simulink model "stuPlutoRx"  (R2021a)
settings: Solver=VariableStepAuto  StartTime=0.0  StopTime=2  RelTol=1e-3
undefined symbols (not defined in the file or in its folder): designMultirateFIR, Fs, ip, usb
libraries: plutoradiolib x1, dsparch4 x1, dspmlti4 x1, dspfdesign x1, dspsrcs4 x1
settings Model: Creator=dm  LastModifiedBy=timingyang
settings SolverCC: AlgebraicLoopSolver=TrustRegion

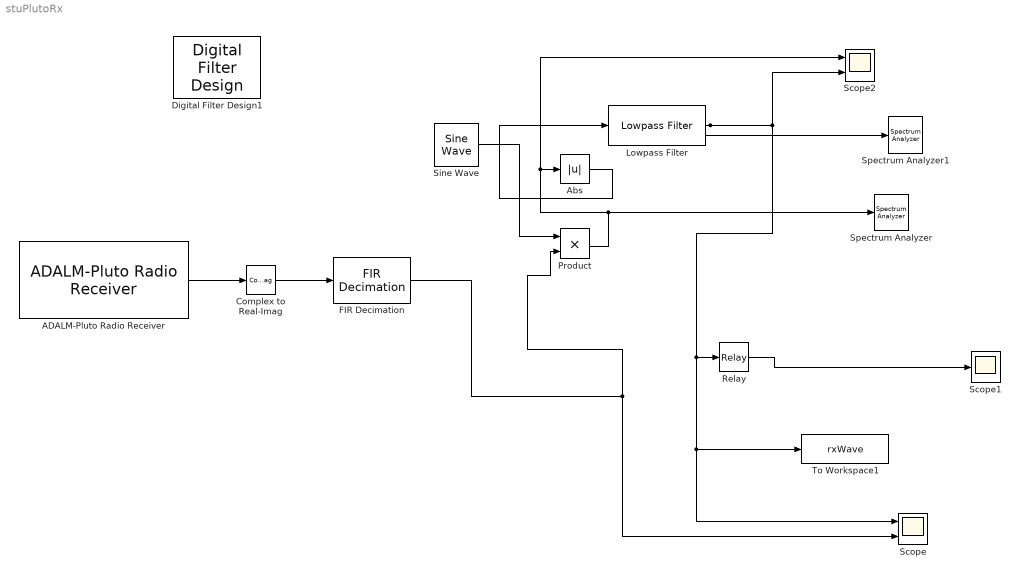
== system stuPlutoRx ==
  ADALM-Pluto Radio Receiver : plutoradiolib/ADALM-Pluto Radio Receiver  RadioID=usb:0  uri=ip:10.0.0.200  CenterFrequencySource=Dialog  CenterFrequency=915.432e6  GainSource=AGC Slow Attack  GainSourceBlock=AGC Slow Attack  Gain=10  ChannelMapping=1  BasebandSampleRate=1e6  OutputDataType=double  SamplesPerFrame=2e4  OverflowOutputPort=off  EnableBurstMode=off  NumFramesInBurst=1  ShowAdvancedProperties=off  UseCustomFilter=off  filtPathRates=[737280000 11520000 3840000 1920000 960000 240000]  filtCoefficients=[-192 82 85 -215 228 -102 -110 290 -318 145 160 -426 471 -215 -238 633 -697 318 349 -923 1009 -457 -498 1309 -1423 640 693 -1812 1959 -876 -945 2458 -2647 1180 1268 -3290 3534 -1572 -1688 4375 -4698 2091 2247 -5836 6284 -2807 -3031 7918 -8588 3870 4225 -11182 12324 -5662 -6330 17255 -19735 9507 11312 -33568 43355 -25227 -42139 305542 305542 -42139 -25227 43355 -33568 11312 9507 -19735 17255 -6330 -5662 12324 -11182 4225 3870 -8588 7918 -3031 -2807 6284 -5836 2247 2091 -4698 4375 -1688 -1572 3534 -3290 1268 1180 -2647 2458 -945 -876 1959 -1812 693 640 -1423 1309 -498 -457 1009 -923 349 318 -697 633 -238 -215 471 -426 160 145 -318 290 -110 -102 228 -215 85 82 -192]  filtCoefficientSize=128  filtDecimInterpFactor=4  filtGain=-12  filtRFBandwidth=18000000  filterConfigStruct=struct()  EnableQuadratureCorrection=on  EnableRFDCCorrection=on  EnableBasebandDCCorrection=on  FrequencyCorrection=0  OverrideSampleTime=off  SampleTime=0.02  DataTimeout=Inf  ENSMPinControlMode=None  BISTLoopbackMode=Disabled  BISTToneInject=Disabled  BISTSignalGen=PRBS  BISTToneFreq=Fs/32  BISTToneLevel=0
      settings: SourceProductBaseCode=PLUTO
  Abs : Abs
  Complex to Real-Imag : ComplexToRealImag  Output=Real
  Digital Filter Design1 : dsparch4/Digital Filter Design  mwdsp_browser_bugfix_var=off
  FIR Decimation : dspmlti4/FIR Decimation  FilterSource=Auto  h=designMultirateFIR(1,2)  D=10  filtStruct=Direct form  FilterObject=FDECIM  InputProcessing=Columns as channels (frame based)  framing=Allow multirate processing  inputOffset=0  outputBufInitCond=0  roundingMode=Floor  overflowMode=off  firstCoeffDataTypeStr=Inherit: Same word length as input  firstCoeffMin=[]  firstCoeffMax=[]  firstCoeffLastDataTypeStr=Inherit: Same word length as input  outputDataTypeStr=Inherit: Same as accumulator  outputMin=[]  outputMax=[]  outputLastDataTypeStr=Inherit: Same as accumulator
  Lowpass Filter : dspfdesign/Lowpass Filter  FilterType=IIR  DesignForMinimumOrder=on  FilterOrder=50  PassbandFrequency=1000  StopbandFrequency=2000  PassbandRipple=0.1  StopbandAttenuation=60  InheritSampleRate=on  SampleRate=44100  SimulateUsing=Interpreted execution  roundingMode=Floor  coeffsDataTypeStr=fixdt(1,16)
  Product : Product
  Relay : Relay  OnSwitchValue=0.05  OffSwitchValue=0.05
  Scope : Scope  NumInputPorts=2
  Scope1 : Scope
  Scope2 : Scope  NumInputPorts=2
  Sine Wave : dspsrcs4/Sine Wave  Amplitude=1  Frequency=10000  Phase=0  SampleMode=Discrete  OutComplex=Real  CompMethod=Trigonometric fcn  TableSize=Speed  SampleTime=1/100e3  SamplesPerFrame=20000  ResetState=Restart at time zero  OutputFrames=off  dataType=double  wordLen=16  udDataType=sfix(16)  fracBitsMode=Best precision  numFracBits=15  OutDataTypeStr=double  LastOutDataTypeStr=double
  Spectrum Analyzer : SpectrumAnalyzer
  Spectrum Analyzer1 : SpectrumAnalyzer
  To Workspace1 : ToWorkspace  VariableName=rxWave  SampleTime=1e-5
      settings: MaxDataPoints=1e5  Decimation=1e4
  wires:
  ADALM-Pluto Radio Receiver/1 -> Complex to Real-Imag/1
  Complex to Real-Imag/1 -> FIR Decimation/1
  Relay/1 -> Scope1/1
  Product/1 -> Scope2/1, Abs/1, Spectrum Analyzer/1
  Sine Wave/1 -> Product/1
  FIR Decimation/1 -> Scope/2, Product/2
  Lowpass Filter/1 -> Spectrum Analyzer1/1, Scope2/2, To Workspace1/1, Scope/1, Relay/1
  Abs/1 -> Lowpass Filter/1
